simulink model "BallScrewModel"  (R2025b)
settings: Solver=VariableStepAuto  StartTime=0.0  StopTime=10.0  RelTol=1e-3
settings Model: Creator=kylea  LastModifiedBy=kylea

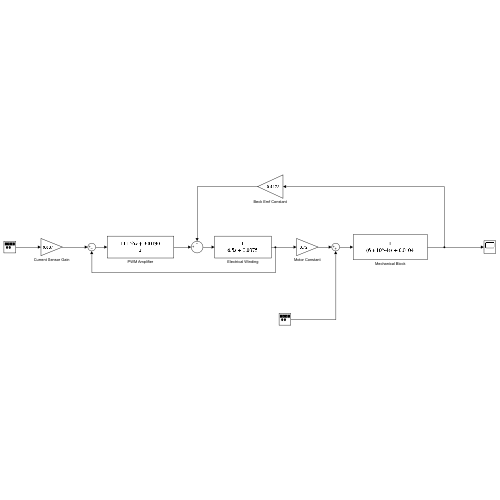
[thumbnail: Simulink's stored preview of the top-level diagram]
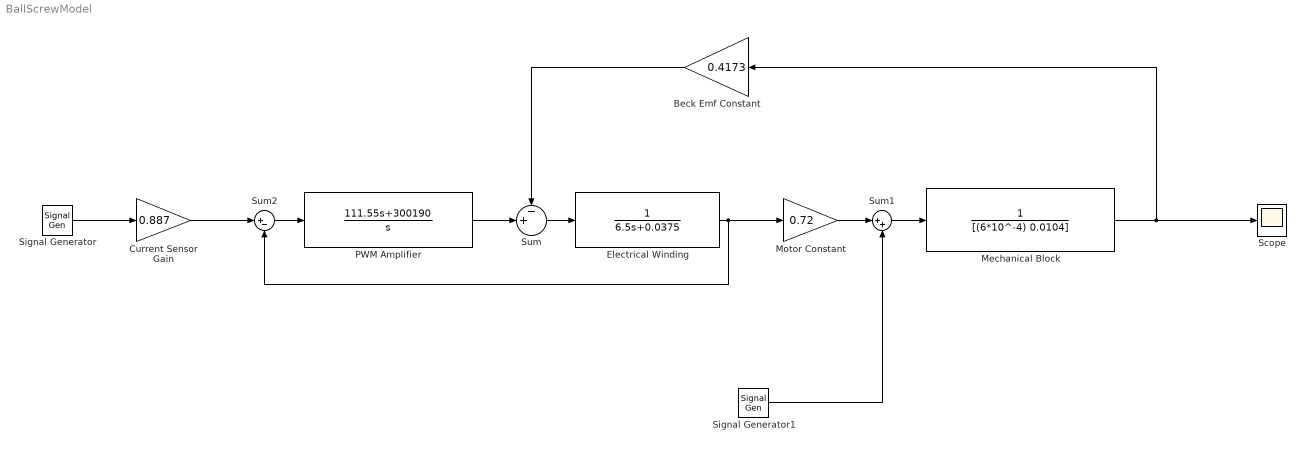
== system BallScrewModel ==
  Beck Emf Constant : Gain  Gain=0.4173
  Current Sensor Gain : Gain  Gain=0.887
  Electrical Winding : TransferFcn  Denominator=[6.5 0.0375]
  Mechanical Block : TransferFcn  Denominator=[(6*10^-4) 0.0104]
  Motor Constant : Gain  Gain=0.72
  PWM Amplifier : TransferFcn  Numerator=[111.55 300190]  Denominator=[1 0]
  Scope : Scope
      settings: ActiveDisplayYMinimum=-196.63438781612084  ActiveDisplayYMaximum=196.63420091342388
  Signal Generator : SignalGenerator  Units=rad/sec
  Signal Generator1 : SignalGenerator  Units=rad/sec
  Sum : Sum  Inputs=-+|
  Sum1 : Sum  Inputs=|++
  Sum2 : Sum  Inputs=|+-
  wires:
  Sum2/1 -> PWM Amplifier/1
  Electrical Winding/1 -> Motor Constant/1, Sum2/2
  Motor Constant/1 -> Sum1/1
  Sum1/1 -> Mechanical Block/1
  Signal Generator/1 -> Current Sensor Gain/1
  Mechanical Block/1 -> Beck Emf Constant/1, Scope/1
  Signal Generator1/1 -> Sum1/2
  Sum/1 -> Electrical Winding/1
  PWM Amplifier/1 -> Sum/2
  Beck Emf Constant/1 -> Sum/1
  Current Sensor Gain/1 -> Sum2/1
